simulink model "PARTE2_sim_gdmc"  (R2020a)
settings: Solver=VariableStepAuto  StartTime=0.0  StopTime=tsim  RelTol=1e-3
values from neighbouring files (symbols this model uses):
  Ts = 1    [PARTE1_gdmc.m]    (also in PARTE2_gdmc_ordem_2.m; PARTE3_gdmc_Nf_20.m; PARTE3_gdmc_Nf_40.m; PARTE4_gdmc_zf_05.m)
undefined symbols (not defined in the file or in its folder): gdmc_simulink
libraries: cstblocks x2, simulink x1
settings Model: Creator=Usuário  LastModifiedBy=Pichau

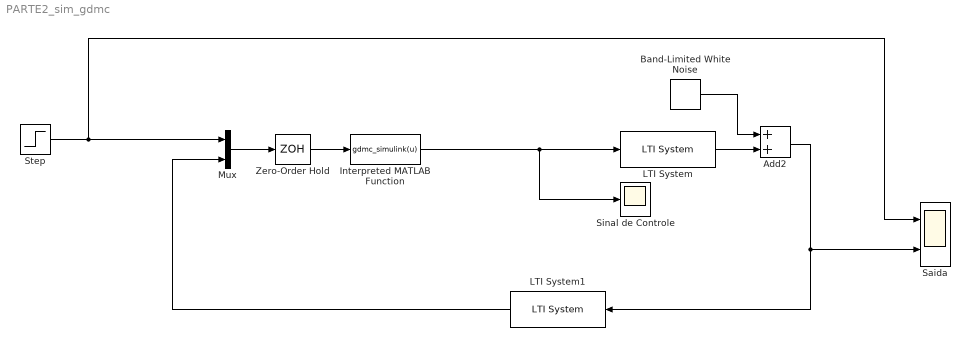
== system PARTE2_sim_gdmc ==
  Add2 : Sum
  Band-Limited White Noise : simulink/Sources/Band-Limited White Noise  Cov=[0.000001]  Ts=0.001  seed=[23341]
  Interpreted MATLAB Function : MATLABFcn  MATLABFcn=gdmc_simulink(u)  OutputDimensions=1
  LTI System : cstblocks/LTI System  sys=Gs  IC=[]
  LTI System1 : cstblocks/LTI System  sys=F  IC=[]
  Mux : Mux  Inputs=2
  Saida : Scope  NumInputPorts=2
  Sinal de Controle : Scope
  Step : Step  Time=4*Ts  SampleTime=0
  Zero-Order Hold : ZeroOrderHold  SampleTime=Ts
  wires:
  Interpreted MATLAB Function/1 -> LTI System/1, Sinal de Controle/1
  Step/1 -> Saida/1, Mux/1
  LTI System/1 -> Add2/2
  Band-Limited White Noise/1 -> Add2/1
  Add2/1 -> Saida/2, LTI System1/1
  LTI System1/1 -> Mux/2
  Mux/1 -> Zero-Order Hold/1
  Zero-Order Hold/1 -> Interpreted MATLAB Function/1
